simulink model "gm_hdl_model_fixed"  (R2024a)
settings: Solver=FixedStepDiscrete  StartTime=0.0  StopTime=SIM_TIME  RelTol=1e-3
undefined symbols (not defined in the file or in its folder): a, b, BUFFER_LEN, c, SAMPLING_FREQ, signal_1
libraries: hdlsllib x39, dspsigops x15, simulink_extras x4, simulink x2, dspsrcs4 x1, dsphdlxfrm2 x1
(part 2 of 3)

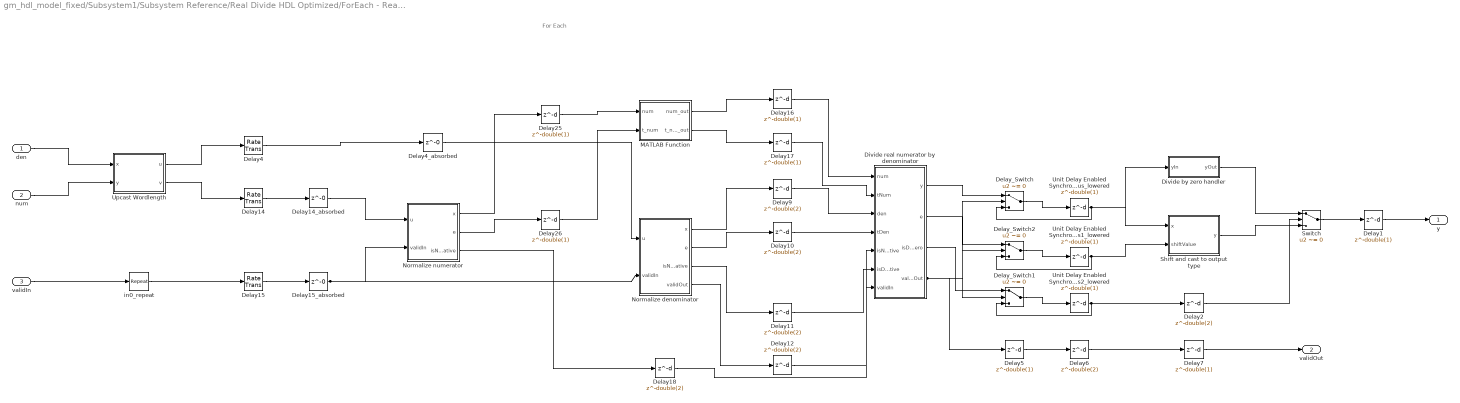
== system gm_hdl_model_fixed/Subsystem1/Subsystem Reference/Real Divide HDL Optimized/ForEach - Real Divide_instance1 ==
  note: For Each
  den : Inport  OutDataTypeStr=fixdt(1, 17, 14)  PortDimensions=1  SampleTime=5e-09
  num : Inport  Port=2  OutDataTypeStr=fixdt(1, 17, 14)  PortDimensions=1  SampleTime=5e-09
  validIn : Inport  Port=3  OutDataTypeStr=boolean  PortDimensions=1  SampleTime=1e-08
  Delay{1,5,7,16..17,25..26} (7 alike) : Delay  DelayLength=double(1)  InitialCondition=0  SampleTime=1e-08
  Delay{2,6,9..12,18} (7 alike) : Delay  DelayLength=double(2)  InitialCondition=0  SampleTime=1e-08
  Delay14 : RateTransition  OutPortSampleTimeOpt=Multiple of input port sample time  OutPortSampleTimeMultiple=2
  Delay14_absorbed : Delay  DelayLength=0
  Delay15 : RateTransition  OutPortSampleTimeOpt=Multiple of input port sample time  OutPortSampleTimeMultiple=2
  Delay15_absorbed : Delay  DelayLength=0
  Delay4 : RateTransition  OutPortSampleTimeOpt=Multiple of input port sample time  OutPortSampleTimeMultiple=2
  Delay4_absorbed : Delay  DelayLength=0
  Delay_Switch : Switch  Criteria=u2 ~= 0  Threshold=double(0)  OutDataTypeStr=fixdt(1, 17, 15)  SampleTime=1e-08  SaturateOnIntegerOverflow=off  InputSameDT=off
  Delay_Switch1 : Switch  Criteria=u2 ~= 0  Threshold=double(0)  OutDataTypeStr=boolean  SampleTime=1e-08  SaturateOnIntegerOverflow=off  InputSameDT=off
  Delay_Switch2 : Switch  Criteria=u2 ~= 0  Threshold=double(0)  OutDataTypeStr=fixdt(1, 34, 0)  SampleTime=1e-08  SaturateOnIntegerOverflow=off  InputSameDT=off
  Divide by zero handler : Subsystem
  Divide real numerator by denominator : Subsystem
  MATLAB Function : Subsystem
  Normalize denominator : Subsystem  mask(Real Normalizer HDL Optimized){}
      mask help: fixed:emblib:RealNormalizerFullDescription
      mask Help: For internal use only. This feature is intentionally undocumented. Its behavior may change, or it may be removed in a future release.
      mask Display:
      | text(0.5,0.8,'u ~= 0','texmode','on','HorizontalAlignment','center')
      | text(0.5,0.6,'x = 2^e |u|','texmode','on','HorizontalAlignment','center')
      | text(0.5,0.4,'1 \leq x < 2','texmode','on','HorizontalAlignment','center')
      | text(0.5,0.2,'isNegative = u<0','texmode','on','HorizontalAlignment','center')
  Normalize numerator : Subsystem  mask(Real Normalizer HDL Optimized){}
      mask help: fixed:emblib:RealNormalizerFullDescription
      mask Help: For internal use only. This feature is intentionally undocumented. Its behavior may change, or it may be removed in a future release.
      mask Display:
      | text(0.5,0.8,'u ~= 0','texmode','on','HorizontalAlignment','center')
      | text(0.5,0.6,'x = 2^e |u|','texmode','on','HorizontalAlignment','center')
      | text(0.5,0.4,'1 \leq x < 2','texmode','on','HorizontalAlignment','center')
      | text(0.5,0.2,'isNegative = u<0','texmode','on','HorizontalAlignment','center')
  Shift and cast to output type : Subsystem  mask{OutputType=OutputType}
      mask prompts: OutputType "fixed:emblib:OutputPrototype"
  Switch : Switch  Criteria=u2 ~= 0  Threshold=double(0)  OutDataTypeStr=fixdt(1, 18, 10)  SampleTime=1e-08  SaturateOnIntegerOverflow=off  InputSameDT=off
  Unit Delay Enabled Synchronous1_lowered : Delay  DelayLength=double(1)  InitialCondition=0  SampleTime=1e-08
  Unit Delay Enabled Synchronous2_lowered : Delay  DelayLength=double(1)  InitialCondition=0  SampleTime=1e-08
  Unit Delay Enabled Synchronous_lowered : Delay  DelayLength=double(1)  InitialCondition=0  SampleTime=1e-08
  Upcast Wordlength : Subsystem
  in0_repeat : dspsigops/Repeat  FactorSource=Dialog parameter  N=double(2)  Nmax=16  RateOptions=Allow multirate processing  ic=0  mode=Unused parameter value
  y : Outport  SampleTime=1e-08
  validOut : Outport  Port=2  SampleTime=1e-08
  wires:
  validIn/1 -> in0_repeat/1
  Shift and cast to output type/1(y) -> Switch/3
  Normalize numerator/1(x) -> Delay25/1
  Normalize numerator/2(e) -> Delay26/1
  Normalize numerator/3(isNegative) -> Delay18/1
  Normalize denominator/1(x) -> Delay9/1
  Normalize denominator/2(e) -> Delay10/1
  Normalize denominator/3(isNegative) -> Delay11/1
  Normalize denominator/4(validOut) -> Delay12/1
  Divide real numerator by denominator/1(y) -> Delay_Switch/1
  Divide real numerator by denominator/2(e) -> Delay_Switch2/1
  Divide real numerator by denominator/3(isDenZero) -> Delay_Switch1/1
  Divide real numerator by denominator/4(validOut) -> Delay5/1, Delay_Switch/2, Delay_Switch1/2, Delay_Switch2/2
  Divide by zero handler/1(yOut) -> Switch/1
  Delay7/1 -> validOut/1
  Delay1/1 -> y/1
  Delay9/1 -> Divide real numerator by denominator/3(den)
  Delay18/1 -> Divide real numerator by denominator/5(isNumNegative)
  Delay12/1 -> Divide real numerator by denominator/7(validIn)
  Delay11/1 -> Divide real numerator by denominator/6(isDenNegative)
  Delay10/1 -> Divide real numerator by denominator/4(tDen)
  Delay16/1 -> Divide real numerator by denominator/1(num)
  Delay17/1 -> Divide real numerator by denominator/2(tNum)
  Delay6/1 -> Delay7/1
  Delay2/1 -> Switch/2
  Delay5/1 -> Delay6/1
  Delay25/1 -> MATLAB Function/1(num)
  Delay26/1 -> MATLAB Function/2(t_num)
  Switch/1 -> Delay1/1
  MATLAB Function/1(num_out) -> Delay16/1
  MATLAB Function/2(t_num_out) -> Delay17/1
  den/1 -> Upcast Wordlength/1(x)
  num/1 -> Upcast Wordlength/2(y)
  Delay15_absorbed/1 -> Normalize denominator/2(validIn), Normalize numerator/2(validIn)
  in0_repeat/1 -> Delay15/1
  Upcast Wordlength/1(u) -> Delay4/1
  Upcast Wordlength/2(v) -> Delay14/1
  Delay4/1 -> Delay4_absorbed/1
  Delay14/1 -> Delay14_absorbed/1
  Delay4_absorbed/1 -> Normalize denominator/1(u)
  Delay14_absorbed/1 -> Normalize numerator/1(u)
  Unit Delay Enabled Synchronous1_lowered/1 -> Delay_Switch2/3, Shift and cast to output type/2(shiftValue)
  Delay_Switch2/1 -> Unit Delay Enabled Synchronous1_lowered/1
  Unit Delay Enabled Synchronous_lowered/1 -> Delay_Switch/3, Divide by zero handler/1(yIn), Shift and cast to output type/1(x)
  Delay_Switch/1 -> Unit Delay Enabled Synchronous_lowered/1
  Unit Delay Enabled Synchronous2_lowered/1 -> Delay_Switch1/3, Delay2/1
  Delay_Switch1/1 -> Unit Delay Enabled Synchronous2_lowered/1
  Delay15/1 -> Delay15_absorbed/1

== system gm_hdl_model_fixed/Subsystem1/Subsystem Reference/Real Divide HDL Optimized/Reshape to original size ==
  y : Inport  OutDataTypeStr=fixdt(1, 18, 10)  PortDimensions=1  SampleTime=1e-08
  u : Inport  Port=2  OutDataTypeStr=fixdt(1, 17, 14)  PortDimensions=1  SampleTime=1e-08
  delayMatch : Delay  DelayLength=double(1)  InitialCondition=0  SampleTime=1e-08
  embreciprocals_c11_Reshape_to_original_size : MATLAB Function  TreatAsAtomicUnit=on
      settings: LibrarySourceBlock=embreciprocals/Real Divide HDL Optimized/Reshape to original size
  z : Outport  SampleTime=1e-08
  wires:
  y/1 -> embreciprocals_c11_Reshape_to_original_size/1(y)
  delayMatch/1 -> embreciprocals_c11_Reshape_to_original_size/2(u)
  embreciprocals_c11_Reshape_to_original_size/1(z) -> z/1
  u/1 -> delayMatch/1

== system gm_hdl_model_fixed/Subsystem1/Subsystem Reference/Real Divide HDL Optimized/Verify divide sizes ==
  denominator : Inport  OutDataTypeStr=fixdt(1, 17, 14)  PortDimensions=1  SampleTime=5e-09
  numerator : Inport  Port=2  OutDataTypeStr=fixdt(1, 17, 14)  PortDimensions=1  SampleTime=5e-09
  delayMatch : Delay  DelayLength=double(3)  InitialCondition=0  SampleTime=5e-09
  embreciprocals_c19_Verify_divide_sizes : MATLAB Function  TreatAsAtomicUnit=on
      settings: LibrarySourceBlock=embreciprocals/Real Divide HDL Optimized/Verify divide sizes
  den : Outport  SampleTime=5e-09
  num : Outport  Port=2  SampleTime=5e-09
  wires:
  denominator/1 -> embreciprocals_c19_Verify_divide_sizes/1(denominator)
  delayMatch/1 -> embreciprocals_c19_Verify_divide_sizes/2(numerator)
  embreciprocals_c19_Verify_divide_sizes/1(den) -> den/1
  embreciprocals_c19_Verify_divide_sizes/2(num) -> num/1
  numerator/1 -> delayMatch/1

== system gm_hdl_model_fixed/Subsystem1/Subsystem Reference/Real Divide HDL Optimized/y = u(1) ==
  u : Inport  OutDataTypeStr=boolean  PortDimensions=1  SampleTime=1e-08
  embreciprocals_c16_y___u_1_ : MATLAB Function  TreatAsAtomicUnit=on
      settings: LibrarySourceBlock=embreciprocals/Real Divide HDL Optimized/y = u(1)
  y : Outport  SampleTime=1e-08
  wires:
  u/1 -> embreciprocals_c16_y___u_1_/1(u)
  embreciprocals_c16_y___u_1_/1(y) -> y/1

== system gm_hdl_model_fixed/Subsystem1/Subsystem Reference/Select_Freq/HDL Counter_controlled ==
  in0 : Inport  OutDataTypeStr=fixdt(0, 12, 0)  SampleTime=1e-08
  stateControl : EnablePort  OutDataTypeStr=boolean
  HDL Counter : Delay  DelayLength=double(1)  InitialCondition=0  SampleTime=1e-08
  out0 : Outport  OutDataTypeStr=fixdt(0, 12, 0)  SampleTime=1e-08
  wires:
  HDL Counter/1 -> out0/1
  in0/1 -> HDL Counter/1

== system gm_hdl_model_fixed/Subsystem1/myRMS/CORDIC Square Root HDL Optimized/Bit Shift Arithmetic ==
  u : Inport  OutDataTypeStr=fixdt(1, 24, 14)  PortDimensions=1  SampleTime=1e-08
  e : Inport  Port=2  OutDataTypeStr=int32  PortDimensions=1  SampleTime=1e-08
  isZero : Inport  Port=3  OutDataTypeStr=boolean  PortDimensions=1  SampleTime=1e-08
  embmathops_c6_st99WwhDyWfnOmuPiiKPkxE_Bit_Shift_Arithmetic : MATLAB Function  TreatAsAtomicUnit=on
      settings: LibrarySourceBlock=embmathops/CORDIC Square Root HDL Optimized/Bit Shift Arithmetic
  y : Outport  SampleTime=1e-08  VectorParamsAs1DForOutWhenUnconnected=off
  wires:
  u/1 -> embmathops_c6_st99WwhDyWfnOmuPiiKPkxE_Bit_Shift_Arithmetic/1(u)
  e/1 -> embmathops_c6_st99WwhDyWfnOmuPiiKPkxE_Bit_Shift_Arithmetic/2(e)
  isZero/1 -> embmathops_c6_st99WwhDyWfnOmuPiiKPkxE_Bit_Shift_Arithmetic/3(isZero)
  embmathops_c6_st99WwhDyWfnOmuPiiKPkxE_Bit_Shift_Arithmetic/1(y) -> y/1

== system gm_hdl_model_fixed/Subsystem1/myRMS/CORDIC Square Root HDL Optimized/Cast to Union of Types ==
  Xref : Inport  OutDataTypeStr=fixdt(0, 16, 7)  SampleTime=1e-08
  Cin : Inport  Port=2  OutDataTypeStr=fixdt(1, 16, 14)  SampleTime=1e-08
  slutils_c1_sjX4rJHbVvOr6YSpugZXv9B_Cast_to_Union_of_Types : MATLAB Function
      settings: LibrarySourceBlock=slutils/Cast to Union of Types
  Cout : Outport  SampleTime=1e-08
  wires:
  Xref/1 -> slutils_c1_sjX4rJHbVvOr6YSpugZXv9B_Cast_to_Union_of_Types/1(Xref)
  Cin/1 -> slutils_c1_sjX4rJHbVvOr6YSpugZXv9B_Cast_to_Union_of_Types/2(Cin)
  slutils_c1_sjX4rJHbVvOr6YSpugZXv9B_Cast_to_Union_of_Types/1(Cout) -> Cout/1

== system gm_hdl_model_fixed/Subsystem1/myRMS/CORDIC Square Root HDL Optimized/Synchronous Subsystem ==
  u : Inport  OutDataTypeStr=fixdt(0, 16, 7)  PortDimensions=1  SampleTime=1e-08
  validIn : Inport  Port=2  OutDataTypeStr=boolean  PortDimensions=1  SampleTime=1e-08
  restart : Inport  Port=3  OutDataTypeStr=boolean  PortDimensions=1  SampleTime=1e-08
  StateControl : StateControl  StateControl=Synchronous
  cordicSquareRootHDL : Subsystem
  dataOut : Outport  SampleTime=1e-08  VectorParamsAs1DForOutWhenUnconnected=off
  eOut : Outport  Port=2  SampleTime=1e-08  VectorParamsAs1DForOutWhenUnconnected=off
  isZero : Outport  Port=3  SampleTime=1e-08  VectorParamsAs1DForOutWhenUnconnected=off
  validOut : Outport  Port=4  SampleTime=1e-08  VectorParamsAs1DForOutWhenUnconnected=off
  wires:
  u/1 -> cordicSquareRootHDL/1(u)
  validIn/1 -> cordicSquareRootHDL/2(validIn)
  restart/1 -> cordicSquareRootHDL/3(restart)
  cordicSquareRootHDL/1(dataOut) -> dataOut/1
  cordicSquareRootHDL/2(eOut) -> eOut/1
  cordicSquareRootHDL/3(isZero) -> isZero/1
  cordicSquareRootHDL/4(validOut) -> validOut/1

== system gm_hdl_model_fixed/Subsystem1/Subsystem Reference/Absolute of Complex/CORDIC Square Root HDL Optimized1/Bit Shift Arithmetic ==
  u : Inport  OutDataTypeStr=fixdt(1, 24, 22)  PortDimensions=1  SampleTime=5e-09
  e : Inport  Port=2  OutDataTypeStr=int32  PortDimensions=1  SampleTime=5e-09
  isZero : Inport  Port=3  OutDataTypeStr=boolean  PortDimensions=1  SampleTime=5e-09
  delayMatch : Delay  DelayLength=double(3)  InitialCondition=0  SampleTime=5e-09
  delayMatch1 : Delay  DelayLength=double(3)  InitialCondition=0  SampleTime=5e-09
  embmathops_c6_s5qJlWhB5AyunXvC1Wsa7cH_Bit_Shift_Arithmetic : MATLAB Function  TreatAsAtomicUnit=on
      settings: LibrarySourceBlock=embmathops/CORDIC Square Root HDL Optimized/Bit Shift Arithmetic
  y : Outport  SampleTime=5e-09  VectorParamsAs1DForOutWhenUnconnected=off
  wires:
  u/1 -> embmathops_c6_s5qJlWhB5AyunXvC1Wsa7cH_Bit_Shift_Arithmetic/1(u)
  delayMatch/1 -> embmathops_c6_s5qJlWhB5AyunXvC1Wsa7cH_Bit_Shift_Arithmetic/2(e)
  delayMatch1/1 -> embmathops_c6_s5qJlWhB5AyunXvC1Wsa7cH_Bit_Shift_Arithmetic/3(isZero)
  embmathops_c6_s5qJlWhB5AyunXvC1Wsa7cH_Bit_Shift_Arithmetic/1(y) -> y/1
  e/1 -> delayMatch/1
  isZero/1 -> delayMatch1/1

== system gm_hdl_model_fixed/Subsystem1/Subsystem Reference/Absolute of Complex/CORDIC Square Root HDL Optimized1/Cast to Union of Types ==
  Xref : Inport  OutDataTypeStr=fixdt(1, 24, 22)  SampleTime=5e-09
  Cin : Inport  Port=2  OutDataTypeStr=fixdt(1, 24, 22)  SampleTime=5e-09
  delayMatch : Delay  DelayLength=double(3)  InitialCondition=0  SampleTime=5e-09
  slutils_c1_sJq36p6JfwxqYYDPRgb8M6G_Cast_to_Union_of_Types : MATLAB Function
      settings: LibrarySourceBlock=slutils/Cast to Union of Types
  Cout : Outport  SampleTime=5e-09
  wires:
  Xref/1 -> slutils_c1_sJq36p6JfwxqYYDPRgb8M6G_Cast_to_Union_of_Types/1(Xref)
  delayMatch/1 -> slutils_c1_sJq36p6JfwxqYYDPRgb8M6G_Cast_to_Union_of_Types/2(Cin)
  slutils_c1_sJq36p6JfwxqYYDPRgb8M6G_Cast_to_Union_of_Types/1(Cout) -> Cout/1
  Cin/1 -> delayMatch/1

== system gm_hdl_model_fixed/Subsystem1/Subsystem Reference/Absolute of Complex/CORDIC Square Root HDL Optimized1/Synchronous Subsystem ==
  u : Inport  OutDataTypeStr=fixdt(1, 24, 22)  PortDimensions=1  SampleTime=5e-09
  validIn : Inport  Port=2  OutDataTypeStr=boolean  PortDimensions=1  SampleTime=1e-08
  restart : Inport  Port=3  OutDataTypeStr=boolean  PortDimensions=1  SampleTime=1e-08
  StateControl : StateControl  StateControl=Synchronous
  cordicSquareRootHDL : Subsystem
  dataOut : Outport  SampleTime=1e-08  VectorParamsAs1DForOutWhenUnconnected=off
  eOut : Outport  Port=2  SampleTime=1e-08  VectorParamsAs1DForOutWhenUnconnected=off
  isZero : Outport  Port=3  SampleTime=1e-08  VectorParamsAs1DForOutWhenUnconnected=off
  validOut : Outport  Port=4  SampleTime=1e-08  VectorParamsAs1DForOutWhenUnconnected=off
  wires:
  validIn/1 -> cordicSquareRootHDL/2(validIn)
  restart/1 -> cordicSquareRootHDL/3(restart)
  cordicSquareRootHDL/1(dataOut) -> dataOut/1
  cordicSquareRootHDL/2(eOut) -> eOut/1
  cordicSquareRootHDL/3(isZero) -> isZero/1
  cordicSquareRootHDL/4(validOut) -> validOut/1
  u/1 -> cordicSquareRootHDL/1(u)

== system gm_hdl_model_fixed/Subsystem1/Subsystem Reference/CORDIC Square Root HDL Optimized/Synchronous Subsystem/cordicSquareRootHDL ==
  u : Inport  OutDataTypeStr=fixdt(1, 22, 20)  PortDimensions=1  SampleTime=1e-08
  validIn : Inport  Port=2  OutDataTypeStr=boolean  PortDimensions=1  SampleTime=1e-08
  restart : Inport  Port=3  OutDataTypeStr=boolean  PortDimensions=1  SampleTime=1e-08
  delayMatch : Delay  DelayLength=double(4)  InitialCondition=0  SampleTime=1e-08
  delayMatch1 : Delay  DelayLength=double(4)  InitialCondition=0  SampleTime=1e-08
  embmathops_c2_skVmLPFzLIK224pVNfQB1qF_cordicSquareRootHDL_controlled : Subsystem
  stateControl : Constant  OutDataTypeStr=boolean  SampleTime=1e-08
  dataOut : Outport  SampleTime=1e-08  VectorParamsAs1DForOutWhenUnconnected=off
  eOut : Outport  Port=2  SampleTime=1e-08
  isZero : Outport  Port=3  SampleTime=1e-08
  validOut : Outport  Port=4  SampleTime=1e-08
  wires:
  u/1 -> embmathops_c2_skVmLPFzLIK224pVNfQB1qF_cordicSquareRootHDL_controlled/1(in0)
  validIn/1 -> embmathops_c2_skVmLPFzLIK224pVNfQB1qF_cordicSquareRootHDL_controlled/2(in1)
  delayMatch/1 -> embmathops_c2_skVmLPFzLIK224pVNfQB1qF_cordicSquareRootHDL_controlled/3(in2)
  embmathops_c2_skVmLPFzLIK224pVNfQB1qF_cordicSquareRootHDL_controlled/1(out0) -> dataOut/1
  embmathops_c2_skVmLPFzLIK224pVNfQB1qF_cordicSquareRootHDL_controlled/2(out1) -> eOut/1
  embmathops_c2_skVmLPFzLIK224pVNfQB1qF_cordicSquareRootHDL_controlled/3(out2) -> isZero/1
  embmathops_c2_skVmLPFzLIK224pVNfQB1qF_cordicSquareRootHDL_controlled/4(out3) -> validOut/1
  delayMatch1/1 -> embmathops_c2_skVmLPFzLIK224pVNfQB1qF_cordicSquareRootHDL_controlled/Enable
  restart/1 -> delayMatch/1
  stateControl/1 -> delayMatch1/1

== system gm_hdl_model_fixed/Subsystem1/Subsystem Reference/Real Divide HDL Optimized/ForEach - Real Divide_instance1/Divide by zero handler ==
  yIn : Inport  OutDataTypeStr=fixdt(1, 17, 15)  SampleTime=1e-08
  Compare To Zero : Subsystem  mask(Compare To Zero){relop=>=, OutDataTypeStr=boolean, ZeroCross=on}
      mask prompts: relop "Simulink:masks:Operator_MP"; OutDataTypeStr "Simulink:masks:OutputDataType_MP"; ZeroCross "Simulink:masks:EnableZerocrossingDetection_MP"
      mask help: Simulink:masks:CompareToZero_MD
      mask init:
      | OutDataTypeStr = 'boolean';
      | ZeroCross = 'on';
      | blkName = 'hdl_model_fixed/Subsystem1/Subsystem Reference/Real Divide HDL Optimized/ForEach - Real Divide/Divide by zero handler/Compare\nTo Zero';
      | relop = '>=';
      | setValue = 'boolean';
      mask TypeOptions relop: == | ~= | < | <= | >= | >
      mask TypeOptions OutDataTypeStr: Simulink:masks:uint8 | Simulink:masks:boolean
      mask Callback ZeroCross: sl('zeroCrossEnable', gcbh);
      mask Display: disp([relop,' 0'])
  Constant3 : Constant  Value=-128  OutDataTypeStr=fixdt(1, 18, 10)  SampleTime=1e-08
  Constant4 : Constant  Value=127.9990234375  OutDataTypeStr=fixdt(1, 18, 10)  SampleTime=1e-08
  Delay13 : Delay  DelayLength=double(1)  InitialCondition=0  SampleTime=1e-08
  Delay3 : Delay  DelayLength=double(1)  InitialCondition=0  SampleTime=1e-08
  Switch : Switch  Criteria=u2 > Threshold  Threshold=double(0)  OutDataTypeStr=fixdt(1, 18, 10)  SampleTime=1e-08  SaturateOnIntegerOverflow=off  InputSameDT=off
  yOut : Outport  SampleTime=1e-08
  wires:
  yIn/1 -> Compare To Zero/1(u)
  Delay3/1 -> yOut/1
  Delay13/1 -> Switch/2
  Constant4/1 -> Switch/1
  Constant3/1 -> Switch/3
  Switch/1 -> Delay3/1
  Compare To Zero/1(y) -> Delay13/1

== system gm_hdl_model_fixed/Subsystem1/Subsystem Reference/Real Divide HDL Optimized/ForEach - Real Divide_instance1/Divide real numerator by denominator ==
  num : Inport  OutDataTypeStr=fixdt(1, 17, 15)  SampleTime=1e-08
  tNum : Inport  Port=2  OutDataTypeStr=fixdt(1, 33, 0)  SampleTime=1e-08
  den : Inport  Port=3  OutDataTypeStr=fixdt(1, 17, 15)  SampleTime=1e-08
  tDen : Inport  Port=4  OutDataTypeStr=int32  SampleTime=1e-08
  isNumNegative : Inport  Port=5  OutDataTypeStr=boolean  SampleTime=1e-08
  isDenNegative : Inport  Port=6  OutDataTypeStr=boolean  SampleTime=1e-08
  validIn : Inport  Port=7  OutDataTypeStr=boolean  SampleTime=1e-08
  normalizedCORDICDivide : Subsystem
  y : Outport  SampleTime=1e-08
  e : Outport  Port=2  SampleTime=1e-08
  isDenZero : Outport  Port=3  SampleTime=1e-08
  validOut : Outport  Port=4  SampleTime=1e-08
  wires:
  normalizedCORDICDivide/1(y) -> y/1
  normalizedCORDICDivide/2(t) -> e/1
  normalizedCORDICDivide/3(isDenZeroOut) -> isDenZero/1
  normalizedCORDICDivide/4(validOut) -> validOut/1
  num/1 -> normalizedCORDICDivide/1(num)
  tNum/1 -> normalizedCORDICDivide/3(tNum)
  den/1 -> normalizedCORDICDivide/2(den)
  tDen/1 -> normalizedCORDICDivide/4(tDen)
  isNumNegative/1 -> normalizedCORDICDivide/5(isNumNegative)
  isDenNegative/1 -> normalizedCORDICDivide/6(isDenNegative)
  validIn/1 -> normalizedCORDICDivide/7(validIn)

== system gm_hdl_model_fixed/Subsystem1/Subsystem Reference/Real Divide HDL Optimized/ForEach - Real Divide_instance1/MATLAB Function ==
  num : Inport  OutDataTypeStr=fixdt(1, 17, 15)  PortDimensions=1  SampleTime=1e-08
  t_num : Inport  Port=2  OutDataTypeStr=int32  PortDimensions=1  SampleTime=1e-08
  embreciprocals_c13_MATLAB_Function : MATLAB Function  TreatAsAtomicUnit=on
      settings: LibrarySourceBlock=embreciprocals/Real Divide HDL Optimized/ForEach - Real Divide/MATLAB Function
  num_out : Outport  SampleTime=1e-08
  t_num_out : Outport  Port=2  SampleTime=1e-08
  wires:
  num/1 -> embreciprocals_c13_MATLAB_Function/1(num)
  t_num/1 -> embreciprocals_c13_MATLAB_Function/2(t_num)
  embreciprocals_c13_MATLAB_Function/1(num_out) -> num_out/1
  embreciprocals_c13_MATLAB_Function/2(t_num_out) -> t_num_out/1

== system gm_hdl_model_fixed/Subsystem1/Subsystem Reference/Real Divide HDL Optimized/ForEach - Real Divide_instance1/Normalize denominator ==
  u : Inport  OutDataTypeStr=fixdt(1, 17, 14)  SampleTime=1e-08
  validIn : Inport  Port=2  OutDataTypeStr=boolean  SampleTime=1e-08
  positiveRealNormalizer : Subsystem
  x : Outport  SampleTime=1e-08
  e : Outport  Port=2  SampleTime=1e-08
  isNegative : Outport  Port=3  SampleTime=1e-08
  validOut : Outport  Port=4  SampleTime=1e-08
  wires:
  positiveRealNormalizer/1(x) -> x/1
  positiveRealNormalizer/2(e) -> e/1
  positiveRealNormalizer/3(isNegative) -> isNegative/1
  positiveRealNormalizer/4(validOut) -> validOut/1
  u/1 -> positiveRealNormalizer/1(u)
  validIn/1 -> positiveRealNormalizer/2(validIn)

== system gm_hdl_model_fixed/Subsystem1/Subsystem Reference/Real Divide HDL Optimized/ForEach - Real Divide_instance1/Normalize numerator ==
  u : Inport  OutDataTypeStr=fixdt(1, 17, 14)  SampleTime=1e-08
  validIn : Inport  Port=2  OutDataTypeStr=boolean  SampleTime=1e-08
  positiveRealNormalizer : Subsystem
  positiveRealNormalizer_term3 : Terminator
  x : Outport  SampleTime=1e-08
  e : Outport  Port=2  SampleTime=1e-08
  isNegative : Outport  Port=3  SampleTime=1e-08
  wires:
  positiveRealNormalizer/1(x) -> x/1
  positiveRealNormalizer/2(e) -> e/1
  positiveRealNormalizer/3(isNegative) -> isNegative/1
  u/1 -> positiveRealNormalizer/1(u)
  validIn/1 -> positiveRealNormalizer/2(validIn)
  positiveRealNormalizer/4(validOut) -> positiveRealNormalizer_term3/1

== system gm_hdl_model_fixed/Subsystem1/Subsystem Reference/Real Divide HDL Optimized/ForEach - Real Divide_instance1/Shift and cast to output type ==
  x : Inport  OutDataTypeStr=fixdt(1, 17, 15)  SampleTime=1e-08
  shiftValue : Inport  Port=2  OutDataTypeStr=fixdt(1, 34, 0)  SampleTime=1e-08
  Abs : Abs  SampleTime=1e-08  OutDataTypeStr=int32  SaturateOnIntegerOverflow=off
  Cast to Union of Types : Subsystem
  Constant : Constant  Value=0  OutDataTypeStr=fixdt(1, 18, 10)  SampleTime=1e-08
  Data Type Conversion : DataTypeConversion  OutDataTypeStr=fixdt(1, 18, 10)  SampleTime=1e-08  RndMeth=Floor
  Delay1 : Delay  DelayLength=double(1)  InitialCondition=0  SampleTime=1e-08
  Delay3 : Delay  DelayLength=double(1)  InitialCondition=0  SampleTime=1e-08
  Switch : Switch  Threshold=double(0)  OutDataTypeStr=fixdt(1, 23, 15)  SampleTime=1e-08  SaturateOnIntegerOverflow=off  InputSameDT=off
  Variable Left Shift : Subsystem
  Variable Right Shift : Subsystem
  y : Outport  SampleTime=1e-08
  wires:
  Variable Right Shift/1(y) -> Switch/3
  Variable Left Shift/1(y) -> Switch/1
  Data Type Conversion/1 -> y/1
  x/1 -> Cast to Union of Types/2(Cin)
  shiftValue/1 -> Abs/1, Delay3/1
  Abs/1 -> Variable Right Shift/2(rightShift), Variable Left Shift/2(leftShift)
  Cast to Union of Types/1(Cout) -> Variable Left Shift/1(x), Variable Right Shift/1(x)
  Delay1/1 -> Data Type Conversion/1
  Delay3/1 -> Switch/2
  Switch/1 -> Delay1/1
  Constant/1 -> Cast to Union of Types/1(Xref)

== system gm_hdl_model_fixed/Subsystem1/Subsystem Reference/Real Divide HDL Optimized/ForEach - Real Divide_instance1/Upcast Wordlength ==
  x : Inport  OutDataTypeStr=fixdt(1, 17, 14)  SampleTime=5e-09
  y : Inport  Port=2  OutDataTypeStr=fixdt(1, 17, 14)  SampleTime=5e-09
  slutils_c2_Upcast_Wordlength : MATLAB Function
      settings: LibrarySourceBlock=slutils/Upcast Wordlength
  u : Outport  SampleTime=5e-09
  v : Outport  Port=2  SampleTime=5e-09
  wires:
  x/1 -> slutils_c2_Upcast_Wordlength/1(x)
  y/1 -> slutils_c2_Upcast_Wordlength/2(y)
  slutils_c2_Upcast_Wordlength/1(u) -> u/1
  slutils_c2_Upcast_Wordlength/2(v) -> v/1

== system gm_hdl_model_fixed/Subsystem1/myRMS/CORDIC Square Root HDL Optimized/Synchronous Subsystem/cordicSquareRootHDL ==
  u : Inport  OutDataTypeStr=fixdt(0, 16, 7)  PortDimensions=1  SampleTime=1e-08
  validIn : Inport  Port=2  OutDataTypeStr=boolean  PortDimensions=1  SampleTime=1e-08
  restart : Inport  Port=3  OutDataTypeStr=boolean  PortDimensions=1  SampleTime=1e-08
  delayMatch : Delay  DelayLength=double(2)  InitialCondition=0  SampleTime=1e-08
  delayMatch1 : Delay  DelayLength=double(2)  InitialCondition=0  SampleTime=1e-08
  embmathops_c2_s84XJG1CWMolALoedlonStG_cordicSquareRootHDL_controlled : Subsystem
  stateControl : Constant  OutDataTypeStr=boolean  SampleTime=1e-08
  dataOut : Outport  SampleTime=1e-08  VectorParamsAs1DForOutWhenUnconnected=off
  eOut : Outport  Port=2  SampleTime=1e-08
  isZero : Outport  Port=3  SampleTime=1e-08
  validOut : Outport  Port=4  SampleTime=1e-08
  wires:
  u/1 -> embmathops_c2_s84XJG1CWMolALoedlonStG_cordicSquareRootHDL_controlled/1(in0)
  validIn/1 -> embmathops_c2_s84XJG1CWMolALoedlonStG_cordicSquareRootHDL_controlled/2(in1)
  delayMatch/1 -> embmathops_c2_s84XJG1CWMolALoedlonStG_cordicSquareRootHDL_controlled/3(in2)
  embmathops_c2_s84XJG1CWMolALoedlonStG_cordicSquareRootHDL_controlled/1(out0) -> dataOut/1
  embmathops_c2_s84XJG1CWMolALoedlonStG_cordicSquareRootHDL_controlled/2(out1) -> eOut/1
  embmathops_c2_s84XJG1CWMolALoedlonStG_cordicSquareRootHDL_controlled/3(out2) -> isZero/1
  embmathops_c2_s84XJG1CWMolALoedlonStG_cordicSquareRootHDL_controlled/4(out3) -> validOut/1
  delayMatch1/1 -> embmathops_c2_s84XJG1CWMolALoedlonStG_cordicSquareRootHDL_controlled/Enable
  restart/1 -> delayMatch/1
  stateControl/1 -> delayMatch1/1

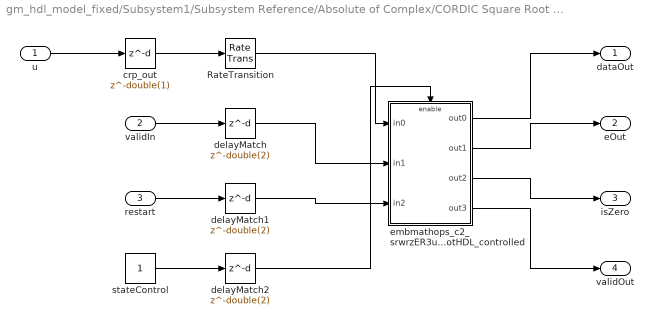
== system gm_hdl_model_fixed/Subsystem1/Subsystem Reference/Absolute of Complex/CORDIC Square Root HDL Optimized1/Synchronous Subsystem/cordicSquareRootHDL ==
  u : Inport  OutDataTypeStr=fixdt(1, 24, 22)  PortDimensions=1  SampleTime=5e-09
  validIn : Inport  Port=2  OutDataTypeStr=boolean  PortDimensions=1  SampleTime=1e-08
  restart : Inport  Port=3  OutDataTypeStr=boolean  PortDimensions=1  SampleTime=1e-08
  RateTransition : RateTransition  OutPortSampleTimeOpt=Multiple of input port sample time  OutPortSampleTimeMultiple=2
  crp_out : Delay  DelayLength=double(1)  InitialCondition=0  SampleTime=5e-09
  delayMatch : Delay  DelayLength=double(2)  InitialCondition=0  SampleTime=1e-08
  delayMatch1 : Delay  DelayLength=double(2)  InitialCondition=0  SampleTime=1e-08
  delayMatch2 : Delay  DelayLength=double(2)  InitialCondition=0  SampleTime=1e-08
  embmathops_c2_srwrzER3uCGRdPfDbow0ID_cordicSquareRootHDL_controlled : Subsystem
  stateControl : Constant  OutDataTypeStr=boolean  SampleTime=1e-08
  dataOut : Outport  SampleTime=1e-08  VectorParamsAs1DForOutWhenUnconnected=off
  eOut : Outport  Port=2  SampleTime=1e-08
  isZero : Outport  Port=3  SampleTime=1e-08
  validOut : Outport  Port=4  SampleTime=1e-08
  wires:
  delayMatch/1 -> embmathops_c2_srwrzER3uCGRdPfDbow0ID_cordicSquareRootHDL_controlled/2(in1)
  delayMatch1/1 -> embmathops_c2_srwrzER3uCGRdPfDbow0ID_cordicSquareRootHDL_controlled/3(in2)
  embmathops_c2_srwrzER3uCGRdPfDbow0ID_cordicSquareRootHDL_controlled/1(out0) -> dataOut/1
  embmathops_c2_srwrzER3uCGRdPfDbow0ID_cordicSquareRootHDL_controlled/2(out1) -> eOut/1
  embmathops_c2_srwrzER3uCGRdPfDbow0ID_cordicSquareRootHDL_controlled/3(out2) -> isZero/1
  embmathops_c2_srwrzER3uCGRdPfDbow0ID_cordicSquareRootHDL_controlled/4(out3) -> validOut/1
  crp_out/1 -> RateTransition/1
  u/1 -> crp_out/1
  RateTransition/1 -> embmathops_c2_srwrzER3uCGRdPfDbow0ID_cordicSquareRootHDL_controlled/1(in0)
  delayMatch2/1 -> embmathops_c2_srwrzER3uCGRdPfDbow0ID_cordicSquareRootHDL_controlled/Enable
  validIn/1 -> delayMatch/1
  restart/1 -> delayMatch1/1
  stateControl/1 -> delayMatch2/1

== system gm_hdl_model_fixed/Subsystem1/Subsystem Reference/CORDIC Square Root HDL Optimized/Synchronous Subsystem/cordicSquareRootHDL/embmathops_c2_skVmLPFzLIK224pVNfQB1qF_cordicSquareRootHDL_controlled ==
  in0 : Inport  OutDataTypeStr=fixdt(1, 22, 20)  SampleTime=1e-08
  in1 : Inport  Port=2  OutDataTypeStr=boolean  SampleTime=1e-08
  in2 : Inport  Port=3  OutDataTypeStr=boolean  SampleTime=1e-08
  stateControl : EnablePort  OutDataTypeStr=boolean
  embmathops_c2_skVmLPFzLIK224pVNfQB1qF_cordicSquareRootHDL : MATLAB Function  TreatAsAtomicUnit=on
      settings: LibrarySourceBlock=embmathops/CORDIC Square Root HDL Optimized/Synchronous Subsystem/cordicSquareRootHDL
  out0 : Outport  OutDataTypeStr=fixdt(1, 22, 20)  SampleTime=1e-08  InitialOutput=0
  out1 : Outport  Port=2  OutDataTypeStr=int32  SampleTime=1e-08  InitialOutput=0
  out2 : Outport  Port=3  OutDataTypeStr=boolean  SampleTime=1e-08  InitialOutput=0
  out3 : Outport  Port=4  OutDataTypeStr=boolean  SampleTime=1e-08  InitialOutput=0
  wires:
  embmathops_c2_skVmLPFzLIK224pVNfQB1qF_cordicSquareRootHDL/1(dataOut) -> out0/1
  embmathops_c2_skVmLPFzLIK224pVNfQB1qF_cordicSquareRootHDL/2(eOut) -> out1/1
  embmathops_c2_skVmLPFzLIK224pVNfQB1qF_cordicSquareRootHDL/3(isZero) -> out2/1
  embmathops_c2_skVmLPFzLIK224pVNfQB1qF_cordicSquareRootHDL/4(validOut) -> out3/1
  in0/1 -> embmathops_c2_skVmLPFzLIK224pVNfQB1qF_cordicSquareRootHDL/1(u)
  in1/1 -> embmathops_c2_skVmLPFzLIK224pVNfQB1qF_cordicSquareRootHDL/2(validIn)
  in2/1 -> embmathops_c2_skVmLPFzLIK224pVNfQB1qF_cordicSquareRootHDL/3(restart)

== system gm_hdl_model_fixed/Subsystem1/Subsystem Reference/Real Divide HDL Optimized/ForEach - Real Divide_instance1/Divide by zero handler/Compare To Zero ==
  u : Inport  OutDataTypeStr=fixdt(1, 17, 15)  SampleTime=1e-08
  Compare : RelationalOperator  OutDataTypeStr=boolean
  Constant : Constant  DisableCoverage=on  Value=0  OutDataTypeStr=fixdt(1, 17, 15)  SampleTime=-1  PreserveConstantTs=on
  y : Outport  SampleTime=1e-08
  wires:
  Constant/1 -> Compare/2
  Compare/1 -> y/1
  u/1 -> Compare/1

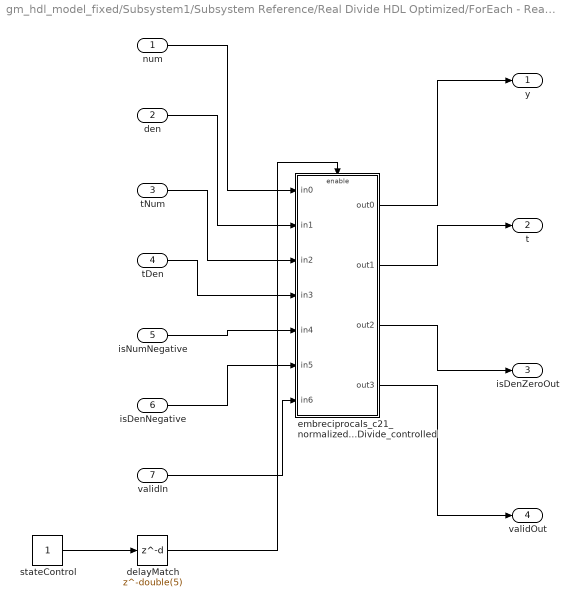
== system gm_hdl_model_fixed/Subsystem1/Subsystem Reference/Real Divide HDL Optimized/ForEach - Real Divide_instance1/Divide real numerator by denominator/normalizedCORDICDivide ==
  num : Inport  OutDataTypeStr=fixdt(1, 17, 15)  PortDimensions=1  SampleTime=1e-08
  den : Inport  Port=2  OutDataTypeStr=fixdt(1, 17, 15)  PortDimensions=1  SampleTime=1e-08
  tNum : Inport  Port=3  OutDataTypeStr=fixdt(1, 33, 0)  PortDimensions=1  SampleTime=1e-08
  tDen : Inport  Port=4  OutDataTypeStr=int32  PortDimensions=1  SampleTime=1e-08
  isNumNegative : Inport  Port=5  OutDataTypeStr=boolean  PortDimensions=1  SampleTime=1e-08
  isDenNegative : Inport  Port=6  OutDataTypeStr=boolean  PortDimensions=1  SampleTime=1e-08
  validIn : Inport  Port=7  OutDataTypeStr=boolean  PortDimensions=1  SampleTime=1e-08
  delayMatch : Delay  DelayLength=double(5)  InitialCondition=0  SampleTime=1e-08
  embreciprocals_c21_normalizedCORDICDivide_controlled : Subsystem
  stateControl : Constant  OutDataTypeStr=boolean  SampleTime=1e-08
  y : Outport  SampleTime=1e-08  VectorParamsAs1DForOutWhenUnconnected=off
  t : Outport  Port=2  SampleTime=1e-08  VectorParamsAs1DForOutWhenUnconnected=off
  isDenZeroOut : Outport  Port=3  SampleTime=1e-08
  validOut : Outport  Port=4  SampleTime=1e-08  VectorParamsAs1DForOutWhenUnconnected=off
  wires:
  num/1 -> embreciprocals_c21_normalizedCORDICDivide_controlled/1(in0)
  den/1 -> embreciprocals_c21_normalizedCORDICDivide_controlled/2(in1)
  tNum/1 -> embreciprocals_c21_normalizedCORDICDivide_controlled/3(in2)
  tDen/1 -> embreciprocals_c21_normalizedCORDICDivide_controlled/4(in3)
  isNumNegative/1 -> embreciprocals_c21_normalizedCORDICDivide_controlled/5(in4)
  isDenNegative/1 -> embreciprocals_c21_normalizedCORDICDivide_controlled/6(in5)
  validIn/1 -> embreciprocals_c21_normalizedCORDICDivide_controlled/7(in6)
  embreciprocals_c21_normalizedCORDICDivide_controlled/1(out0) -> y/1
  embreciprocals_c21_normalizedCORDICDivide_controlled/2(out1) -> t/1
  embreciprocals_c21_normalizedCORDICDivide_controlled/3(out2) -> isDenZeroOut/1
  embreciprocals_c21_normalizedCORDICDivide_controlled/4(out3) -> validOut/1
  delayMatch/1 -> embreciprocals_c21_normalizedCORDICDivide_controlled/Enable
  stateControl/1 -> delayMatch/1

== system gm_hdl_model_fixed/Subsystem1/Subsystem Reference/Real Divide HDL Optimized/ForEach - Real Divide_instance1/Normalize denominator/positiveRealNormalizer ==
  u : Inport  OutDataTypeStr=fixdt(1, 17, 14)  PortDimensions=1  SampleTime=1e-08
  validIn : Inport  Port=2  OutDataTypeStr=boolean  PortDimensions=1  SampleTime=1e-08
  delayMatch : Delay  DelayLength=double(2)  InitialCondition=0  SampleTime=1e-08
  delayMatch1 : Delay  DelayLength=double(5)  InitialCondition=0  SampleTime=1e-08
  embreciprocals_c3_positiveRealNormalizer_controlled : Subsystem
  stateControl : Constant  OutDataTypeStr=boolean  SampleTime=1e-08
  x : Outport  SampleTime=1e-08  VectorParamsAs1DForOutWhenUnconnected=off
  e : Outport  Port=2  SampleTime=1e-08  VectorParamsAs1DForOutWhenUnconnected=off
  isNegative : Outport  Port=3  SampleTime=1e-08
  validOut : Outport  Port=4  SampleTime=1e-08  VectorParamsAs1DForOutWhenUnconnected=off
  wires:
  u/1 -> embreciprocals_c3_positiveRealNormalizer_controlled/1(in0)
  delayMatch/1 -> embreciprocals_c3_positiveRealNormalizer_controlled/2(in1)
  embreciprocals_c3_positiveRealNormalizer_controlled/1(out0) -> x/1
  embreciprocals_c3_positiveRealNormalizer_controlled/2(out1) -> e/1
  embreciprocals_c3_positiveRealNormalizer_controlled/3(out2) -> isNegative/1
  embreciprocals_c3_positiveRealNormalizer_controlled/4(out3) -> validOut/1
  delayMatch1/1 -> embreciprocals_c3_positiveRealNormalizer_controlled/Enable
  validIn/1 -> delayMatch/1
  stateControl/1 -> delayMatch1/1

== system gm_hdl_model_fixed/Subsystem1/Subsystem Reference/Real Divide HDL Optimized/ForEach - Real Divide_instance1/Normalize numerator/positiveRealNormalizer ==
  u : Inport  OutDataTypeStr=fixdt(1, 17, 14)  PortDimensions=1  SampleTime=1e-08
  validIn : Inport  Port=2  OutDataTypeStr=boolean  PortDimensions=1  SampleTime=1e-08
  delayMatch : Delay  DelayLength=double(2)  InitialCondition=0  SampleTime=1e-08
  delayMatch1 : Delay  DelayLength=double(5)  InitialCondition=0  SampleTime=1e-08
  embreciprocals_c3_positiveRealNormalizer_controlled : Subsystem
  embreciprocals_c3_positiveRealNormalizer_controlled_term3 : Terminator
  stateControl : Constant  OutDataTypeStr=boolean  SampleTime=1e-08
  t : Constant  Value=double(0)  OutDataTypeStr=boolean  SampleTime=1e-08
  x : Outport  SampleTime=1e-08  VectorParamsAs1DForOutWhenUnconnected=off
  e : Outport  Port=2  SampleTime=1e-08  VectorParamsAs1DForOutWhenUnconnected=off
  isNegative : Outport  Port=3  SampleTime=1e-08
  validOut : Outport  Port=4  SampleTime=1e-08  VectorParamsAs1DForOutWhenUnconnected=off
  wires:
  u/1 -> embreciprocals_c3_positiveRealNormalizer_controlled/1(in0)
  delayMatch/1 -> embreciprocals_c3_positiveRealNormalizer_controlled/2(in1)
  embreciprocals_c3_positiveRealNormalizer_controlled/1(out0) -> x/1
  embreciprocals_c3_positiveRealNormalizer_controlled/2(out1) -> e/1
  embreciprocals_c3_positiveRealNormalizer_controlled/3(out2) -> isNegative/1
  embreciprocals_c3_positiveRealNormalizer_controlled/4(out3) -> embreciprocals_c3_positiveRealNormalizer_controlled_term3/1
  t/1 -> validOut/1
  delayMatch1/1 -> embreciprocals_c3_positiveRealNormalizer_controlled/Enable
  validIn/1 -> delayMatch/1
  stateControl/1 -> delayMatch1/1

== system gm_hdl_model_fixed/Subsystem1/Subsystem Reference/Real Divide HDL Optimized/ForEach - Real Divide_instance1/Shift and cast to output type/Cast to Union of Types ==
  Xref : Inport  OutDataTypeStr=fixdt(1, 18, 10)  SampleTime=1e-08
  Cin : Inport  Port=2  OutDataTypeStr=fixdt(1, 17, 15)  SampleTime=1e-08
  slutils_c1_sfkclysknIFh6pVVpTDebQG_Cast_to_Union_of_Types : MATLAB Function
      settings: LibrarySourceBlock=slutils/Cast to Union of Types
  Cout : Outport  SampleTime=1e-08
  wires:
  Xref/1 -> slutils_c1_sfkclysknIFh6pVVpTDebQG_Cast_to_Union_of_Types/1(Xref)
  Cin/1 -> slutils_c1_sfkclysknIFh6pVVpTDebQG_Cast_to_Union_of_Types/2(Cin)
  slutils_c1_sfkclysknIFh6pVVpTDebQG_Cast_to_Union_of_Types/1(Cout) -> Cout/1

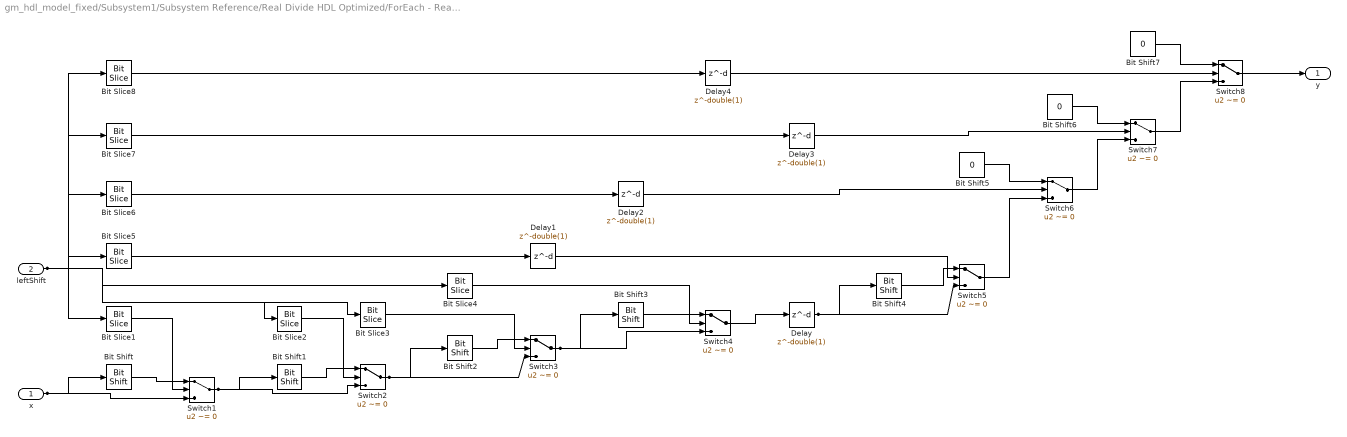
== system gm_hdl_model_fixed/Subsystem1/Subsystem Reference/Real Divide HDL Optimized/ForEach - Real Divide_instance1/Shift and cast to output type/Variable Left Shift ==
  x : Inport  OutDataTypeStr=fixdt(1, 23, 15)  SampleTime=1e-08
  leftShift : Inport  Port=2  OutDataTypeStr=int32  SampleTime=1e-08
  Bit Shift : hdlsllib/Logic and Bit Operations/Bit Shift  mode=Shift Left Logical  N=double(1)
  Bit Shift1 : hdlsllib/Logic and Bit Operations/Bit Shift  mode=Shift Left Logical  N=double(2)
  Bit Shift2 : hdlsllib/Logic and Bit Operations/Bit Shift  mode=Shift Left Logical  N=double(4)
  Bit Shift3 : hdlsllib/Logic and Bit Operations/Bit Shift  mode=Shift Left Logical  N=double(8)
  Bit Shift4 : hdlsllib/Logic and Bit Operations/Bit Shift  mode=Shift Left Logical  N=double(16)
  Bit Shift5 : Constant  Value=0  OutDataTypeStr=fixdt(1, 23, 15)  SampleTime=1e-08
  Bit Shift6 : Constant  Value=0  OutDataTypeStr=fixdt(1, 23, 15)  SampleTime=1e-08
  Bit Shift7 : Constant  Value=0  OutDataTypeStr=fixdt(1, 23, 15)  SampleTime=1e-08
  Bit Slice1 : hdlsllib/Logic and Bit Operations/Bit Slice  lidx=double(0)  ridx=double(0)
  Bit Slice2 : hdlsllib/Logic and Bit Operations/Bit Slice  lidx=double(1)  ridx=double(1)
  Bit Slice3 : hdlsllib/Logic and Bit Operations/Bit Slice  lidx=double(2)  ridx=double(2)
  Bit Slice4 : hdlsllib/Logic and Bit Operations/Bit Slice  lidx=double(3)  ridx=double(3)
  Bit Slice5 : hdlsllib/Logic and Bit Operations/Bit Slice  lidx=double(4)  ridx=double(4)
  Bit Slice6 : hdlsllib/Logic and Bit Operations/Bit Slice  lidx=double(5)  ridx=double(5)
  Bit Slice7 : hdlsllib/Logic and Bit Operations/Bit Slice  lidx=double(6)  ridx=double(6)
  Bit Slice8 : hdlsllib/Logic and Bit Operations/Bit Slice  lidx=double(7)  ridx=double(7)
  Delay{,1..4} (5 alike) : Delay  DelayLength=double(1)  InitialCondition=0  SampleTime=1e-08
  Switch{1..8} (8 alike) : Switch  Criteria=u2 ~= 0  Threshold=double(0)  OutDataTypeStr=fixdt(1, 23, 15)  SampleTime=1e-08  SaturateOnIntegerOverflow=off  InputSameDT=off
  y : Outport  SampleTime=1e-08
  wires:
  Switch8/1 -> y/1
  x/1 -> Switch1/3, Bit Shift/1
  leftShift/1 -> Bit Slice4/1, Bit Slice3/1, Bit Slice2/1, Bit Slice1/1, Bit Slice5/1, Bit Slice6/1, Bit Slice7/1, Bit Slice8/1
  Delay4/1 -> Switch8/2
  Delay3/1 -> Switch7/2
  Delay2/1 -> Switch6/2
  Delay1/1 -> Switch5/2
  Delay/1 -> Switch5/3, Bit Shift4/1
  Bit Shift4/1 -> Switch5/1
  Switch5/1 -> Switch6/3
  Bit Shift5/1 -> Switch6/1
  Switch6/1 -> Switch7/3
  Bit Shift6/1 -> Switch7/1
  Switch7/1 -> Switch8/3
  Bit Shift7/1 -> Switch8/1
  Bit Slice8/1 -> Delay4/1
  Bit Slice7/1 -> Delay3/1
  Bit Slice6/1 -> Delay2/1
  Bit Slice5/1 -> Delay1/1
  Bit Shift/1 -> Switch1/1
  Bit Slice1/1 -> Switch1/2
  Switch1/1 -> Switch2/3, Bit Shift1/1
  Bit Shift1/1 -> Switch2/1
  Bit Slice2/1 -> Switch2/2
  Switch2/1 -> Switch3/3, Bit Shift2/1
  Bit Shift2/1 -> Switch3/1
  Bit Slice3/1 -> Switch3/2
  Switch3/1 -> Switch4/3, Bit Shift3/1
  Bit Shift3/1 -> Switch4/1
  Bit Slice4/1 -> Switch4/2
  Switch4/1 -> Delay/1

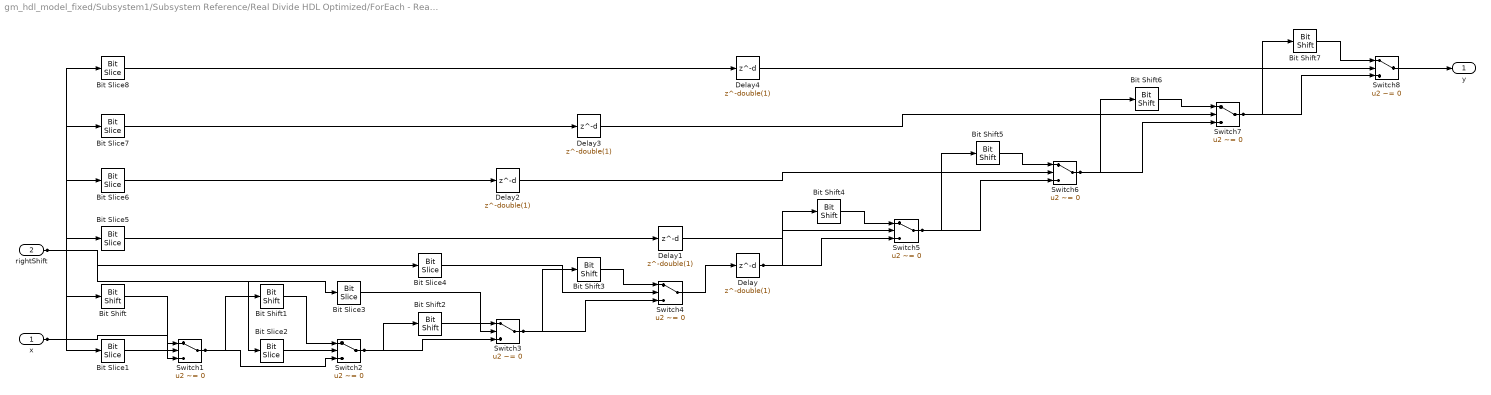
== system gm_hdl_model_fixed/Subsystem1/Subsystem Reference/Real Divide HDL Optimized/ForEach - Real Divide_instance1/Shift and cast to output type/Variable Right Shift ==
  x : Inport  OutDataTypeStr=fixdt(1, 23, 15)  SampleTime=1e-08
  rightShift : Inport  Port=2  OutDataTypeStr=int32  SampleTime=1e-08
  Bit Shift : hdlsllib/Logic and Bit Operations/Bit Shift  mode=Shift Right Arithmetic  N=double(1)
  Bit Shift1 : hdlsllib/Logic and Bit Operations/Bit Shift  mode=Shift Right Arithmetic  N=double(2)
  Bit Shift2 : hdlsllib/Logic and Bit Operations/Bit Shift  mode=Shift Right Arithmetic  N=double(4)
  Bit Shift3 : hdlsllib/Logic and Bit Operations/Bit Shift  mode=Shift Right Arithmetic  N=double(8)
  Bit Shift4 : hdlsllib/Logic and Bit Operations/Bit Shift  mode=Shift Right Arithmetic  N=double(16)
  Bit Shift5 : hdlsllib/Logic and Bit Operations/Bit Shift  mode=Shift Right Arithmetic  N=double(22)
  Bit Shift6 : hdlsllib/Logic and Bit Operations/Bit Shift  mode=Shift Right Arithmetic  N=double(22)
  Bit Shift7 : hdlsllib/Logic and Bit Operations/Bit Shift  mode=Shift Right Arithmetic  N=double(22)
  Bit Slice1 : hdlsllib/Logic and Bit Operations/Bit Slice  lidx=double(0)  ridx=double(0)
  Bit Slice2 : hdlsllib/Logic and Bit Operations/Bit Slice  lidx=double(1)  ridx=double(1)
  Bit Slice3 : hdlsllib/Logic and Bit Operations/Bit Slice  lidx=double(2)  ridx=double(2)
  Bit Slice4 : hdlsllib/Logic and Bit Operations/Bit Slice  lidx=double(3)  ridx=double(3)
  Bit Slice5 : hdlsllib/Logic and Bit Operations/Bit Slice  lidx=double(4)  ridx=double(4)
  Bit Slice6 : hdlsllib/Logic and Bit Operations/Bit Slice  lidx=double(5)  ridx=double(5)
  Bit Slice7 : hdlsllib/Logic and Bit Operations/Bit Slice  lidx=double(6)  ridx=double(6)
  Bit Slice8 : hdlsllib/Logic and Bit Operations/Bit Slice  lidx=double(7)  ridx=double(7)
  Delay{,1..4} (5 alike) : Delay  DelayLength=double(1)  InitialCondition=0  SampleTime=1e-08
  Switch{1..8} (8 alike) : Switch  Criteria=u2 ~= 0  Threshold=double(0)  OutDataTypeStr=fixdt(1, 23, 15)  SampleTime=1e-08  SaturateOnIntegerOverflow=off  InputSameDT=off
  y : Outport  SampleTime=1e-08
  wires:
  Switch8/1 -> y/1
  x/1 -> Switch1/3, Bit Shift/1
  rightShift/1 -> Bit Slice4/1, Bit Slice3/1, Bit Slice2/1, Bit Slice1/1, Bit Slice5/1, Bit Slice6/1, Bit Slice7/1, Bit Slice8/1
  Delay4/1 -> Switch8/2
  Delay3/1 -> Switch7/2
  Delay2/1 -> Switch6/2
  Delay1/1 -> Switch5/2
  Delay/1 -> Switch5/3, Bit Shift4/1
  Bit Shift4/1 -> Switch5/1
  Switch5/1 -> Switch6/3, Bit Shift5/1
  Bit Shift5/1 -> Switch6/1
  Switch6/1 -> Switch7/3, Bit Shift6/1
  Bit Shift6/1 -> Switch7/1
  Switch7/1 -> Switch8/3, Bit Shift7/1
  Bit Shift7/1 -> Switch8/1
  Bit Slice8/1 -> Delay4/1
  Bit Slice7/1 -> Delay3/1
  Bit Slice6/1 -> Delay2/1
  Bit Slice5/1 -> Delay1/1
  Bit Shift/1 -> Switch1/1
  Bit Slice1/1 -> Switch1/2
  Switch1/1 -> Switch2/3, Bit Shift1/1
  Bit Shift1/1 -> Switch2/1
  Bit Slice2/1 -> Switch2/2
  Switch2/1 -> Switch3/3, Bit Shift2/1
  Bit Shift2/1 -> Switch3/1
  Bit Slice3/1 -> Switch3/2
  Switch3/1 -> Switch4/3, Bit Shift3/1
  Bit Shift3/1 -> Switch4/1
  Bit Slice4/1 -> Switch4/2
  Switch4/1 -> Delay/1

== system gm_hdl_model_fixed/Subsystem1/myRMS/CORDIC Square Root HDL Optimized/Synchronous Subsystem/cordicSquareRootHDL/embmathops_c2_s84XJG1CWMolALoedlonStG_cordicSquareRootHDL_controlled ==
  in0 : Inport  OutDataTypeStr=fixdt(0, 16, 7)  SampleTime=1e-08
  in1 : Inport  Port=2  OutDataTypeStr=boolean  SampleTime=1e-08
  in2 : Inport  Port=3  OutDataTypeStr=boolean  SampleTime=1e-08
  stateControl : EnablePort  OutDataTypeStr=boolean
  embmathops_c2_s84XJG1CWMolALoedlonStG_cordicSquareRootHDL : MATLAB Function  TreatAsAtomicUnit=on
      settings: LibrarySourceBlock=embmathops/CORDIC Square Root HDL Optimized/Synchronous Subsystem/cordicSquareRootHDL
  out0 : Outport  OutDataTypeStr=fixdt(1, 16, 14)  SampleTime=1e-08  InitialOutput=0
  out1 : Outport  Port=2  OutDataTypeStr=int32  SampleTime=1e-08  InitialOutput=0
  out2 : Outport  Port=3  OutDataTypeStr=boolean  SampleTime=1e-08  InitialOutput=0
  out3 : Outport  Port=4  OutDataTypeStr=boolean  SampleTime=1e-08  InitialOutput=0
  wires:
  embmathops_c2_s84XJG1CWMolALoedlonStG_cordicSquareRootHDL/1(dataOut) -> out0/1
  embmathops_c2_s84XJG1CWMolALoedlonStG_cordicSquareRootHDL/2(eOut) -> out1/1
  embmathops_c2_s84XJG1CWMolALoedlonStG_cordicSquareRootHDL/3(isZero) -> out2/1
  embmathops_c2_s84XJG1CWMolALoedlonStG_cordicSquareRootHDL/4(validOut) -> out3/1
  in0/1 -> embmathops_c2_s84XJG1CWMolALoedlonStG_cordicSquareRootHDL/1(u)
  in1/1 -> embmathops_c2_s84XJG1CWMolALoedlonStG_cordicSquareRootHDL/2(validIn)
  in2/1 -> embmathops_c2_s84XJG1CWMolALoedlonStG_cordicSquareRootHDL/3(restart)

== system gm_hdl_model_fixed/Subsystem1/Subsystem Reference/Absolute of Complex/CORDIC Square Root HDL Optimized1/Synchronous Subsystem/cordicSquareRootHDL/embmathops_c2_srwrzER3uCGRdPfDbow0ID_cordicSquareRootHDL_controlled ==
  in0 : Inport  OutDataTypeStr=fixdt(1, 24, 22)  SampleTime=1e-08
  in1 : Inport  Port=2  OutDataTypeStr=boolean  SampleTime=1e-08
  in2 : Inport  Port=3  OutDataTypeStr=boolean  SampleTime=1e-08
  stateControl : EnablePort  OutDataTypeStr=boolean
  embmathops_c2_srwrzER3uCGRdPfDbow0ID_cordicSquareRootHDL : MATLAB Function  TreatAsAtomicUnit=on
      settings: LibrarySourceBlock=embmathops/CORDIC Square Root HDL Optimized/Synchronous Subsystem/cordicSquareRootHDL
  out0 : Outport  OutDataTypeStr=fixdt(1, 24, 22)  SampleTime=1e-08  InitialOutput=0
  out1 : Outport  Port=2  OutDataTypeStr=int32  SampleTime=1e-08  InitialOutput=0
  out2 : Outport  Port=3  OutDataTypeStr=boolean  SampleTime=1e-08  InitialOutput=0
  out3 : Outport  Port=4  OutDataTypeStr=boolean  SampleTime=1e-08  InitialOutput=0
  wires:
  embmathops_c2_srwrzER3uCGRdPfDbow0ID_cordicSquareRootHDL/1(dataOut) -> out0/1
  embmathops_c2_srwrzER3uCGRdPfDbow0ID_cordicSquareRootHDL/2(eOut) -> out1/1
  embmathops_c2_srwrzER3uCGRdPfDbow0ID_cordicSquareRootHDL/3(isZero) -> out2/1
  embmathops_c2_srwrzER3uCGRdPfDbow0ID_cordicSquareRootHDL/4(validOut) -> out3/1
  in0/1 -> embmathops_c2_srwrzER3uCGRdPfDbow0ID_cordicSquareRootHDL/1(u)
  in1/1 -> embmathops_c2_srwrzER3uCGRdPfDbow0ID_cordicSquareRootHDL/2(validIn)
  in2/1 -> embmathops_c2_srwrzER3uCGRdPfDbow0ID_cordicSquareRootHDL/3(restart)

== system gm_hdl_model_fixed/Subsystem1/Subsystem Reference/Real Divide HDL Optimized/ForEach - Real Divide_instance1/Divide real numerator by denominator/normalizedCORDICDivide/embreciprocals_c21_normalizedCORDICDivide_controlled ==
  in0 : Inport  OutDataTypeStr=fixdt(1, 17, 15)  SampleTime=1e-08
  in1 : Inport  Port=2  OutDataTypeStr=fixdt(1, 17, 15)  SampleTime=1e-08
  in2 : Inport  Port=3  OutDataTypeStr=fixdt(1, 33, 0)  SampleTime=1e-08
  in3 : Inport  Port=4  OutDataTypeStr=int32  SampleTime=1e-08
  in4 : Inport  Port=5  OutDataTypeStr=boolean  SampleTime=1e-08
  in5 : Inport  Port=6  OutDataTypeStr=boolean  SampleTime=1e-08
  in6 : Inport  Port=7  OutDataTypeStr=boolean  SampleTime=1e-08
  stateControl : EnablePort  OutDataTypeStr=boolean
  embreciprocals_c21_normalizedCORDICDivide : MATLAB Function  TreatAsAtomicUnit=on
      settings: LibrarySourceBlock=embreciprocals/Divide real numerator by denominator/normalizedCORDICDivide
  out0 : Outport  OutDataTypeStr=fixdt(1, 17, 15)  SampleTime=1e-08  InitialOutput=0
  out1 : Outport  Port=2  OutDataTypeStr=fixdt(1, 34, 0)  SampleTime=1e-08  InitialOutput=0
  out2 : Outport  Port=3  OutDataTypeStr=boolean  SampleTime=1e-08  InitialOutput=0
  out3 : Outport  Port=4  OutDataTypeStr=boolean  SampleTime=1e-08  InitialOutput=0
  wires:
  embreciprocals_c21_normalizedCORDICDivide/1(y) -> out0/1
  embreciprocals_c21_normalizedCORDICDivide/2(t) -> out1/1
  embreciprocals_c21_normalizedCORDICDivide/3(isDenZeroOut) -> out2/1
  embreciprocals_c21_normalizedCORDICDivide/4(validOut) -> out3/1
  in0/1 -> embreciprocals_c21_normalizedCORDICDivide/1(num)
  in1/1 -> embreciprocals_c21_normalizedCORDICDivide/2(den)
  in2/1 -> embreciprocals_c21_normalizedCORDICDivide/3(tNum)
  in3/1 -> embreciprocals_c21_normalizedCORDICDivide/4(tDen)
  in4/1 -> embreciprocals_c21_normalizedCORDICDivide/5(isNumNegative)
  in5/1 -> embreciprocals_c21_normalizedCORDICDivide/6(isDenNegative)
  in6/1 -> embreciprocals_c21_normalizedCORDICDivide/7(validIn)

== system gm_hdl_model_fixed/Subsystem1/Subsystem Reference/Real Divide HDL Optimized/ForEach - Real Divide_instance1/Normalize denominator/positiveRealNormalizer/embreciprocals_c3_positiveRealNormalizer_controlled ==
  in0 : Inport  OutDataTypeStr=fixdt(1, 17, 14)  SampleTime=1e-08
  in1 : Inport  Port=2  OutDataTypeStr=boolean  SampleTime=1e-08
  stateControl : EnablePort  OutDataTypeStr=boolean
  embreciprocals_c3_positiveRealNormalizer : MATLAB Function  TreatAsAtomicUnit=on
      settings: LibrarySourceBlock=embreciprocals/Real Normalizer HDL Optimized/positiveRealNormalizer
  out0 : Outport  OutDataTypeStr=fixdt(1, 17, 15)  SampleTime=1e-08  InitialOutput=0
  out1 : Outport  Port=2  OutDataTypeStr=int32  SampleTime=1e-08  InitialOutput=0
  out2 : Outport  Port=3  OutDataTypeStr=boolean  SampleTime=1e-08  InitialOutput=0
  out3 : Outport  Port=4  OutDataTypeStr=boolean  SampleTime=1e-08  InitialOutput=0
  wires:
  embreciprocals_c3_positiveRealNormalizer/1(x) -> out0/1
  embreciprocals_c3_positiveRealNormalizer/2(e) -> out1/1
  embreciprocals_c3_positiveRealNormalizer/3(isNegative) -> out2/1
  embreciprocals_c3_positiveRealNormalizer/4(validOut) -> out3/1
  in0/1 -> embreciprocals_c3_positiveRealNormalizer/1(u)
  in1/1 -> embreciprocals_c3_positiveRealNormalizer/2(validIn)
